simulink model "pv_battery_converter_simulation"  (Simulink 8.8)
settings: Solver=ode45  StartTime=0.0  StopTime=3600*14  FixedStep=0.01  RelTol=1e-3  EnableMultiTasking=on
undefined symbols (not defined in the file): G_vec, Ppv_to_Ipv, Ppv_vec
libraries: simulink x2
settings Model: LogicAnalyzerSignalOrdering=50bcff72-ad36-4fbe-b64f-51c65f6cd540,5d435876-f604-47e5-bfe3-cb9cb4b23e1d,6b0e0226-71fb-4e57-ad2a-fabfdac615dd,e2076062-044c-4264-af36-cff1764121ec,6ceae382-cfb6-4c2b-9ce8-e51f041ad3d8,832e4e12-eea1-4e74-bd4f-841bea17a355,4353c241-6b25-4e3c-9a1f-18ea053f432e  SuppressorTable=22 serialization::archive 11 0 3 0 0 0 0 0  Creator=dhshin  LastModifiedBy=Robert
settings OptimizationCC: ExpressionDepthLimit=2147483647
settings DebuggingCC: SolverPrmCheckMsg=warning

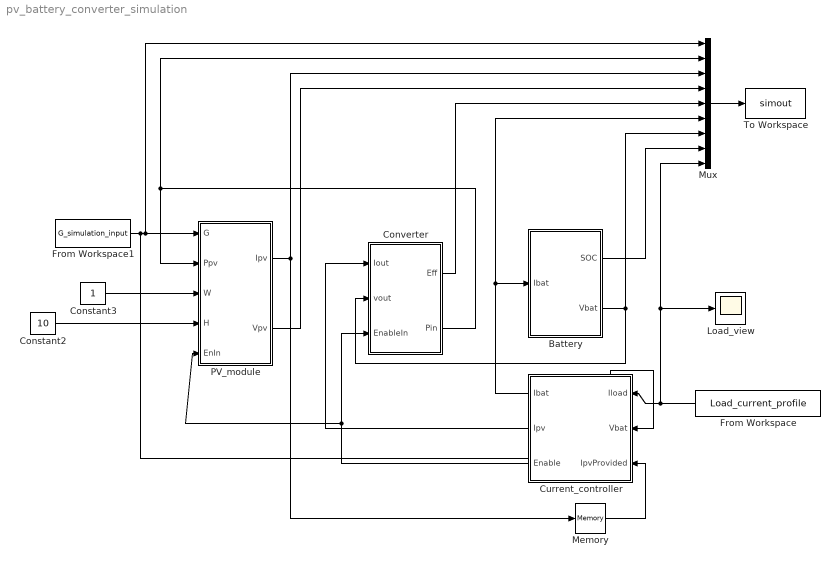
== system pv_battery_converter_simulation ==
  Battery : Subsystem
  Constant2 : Constant  Value=10
  Constant3 : Constant
  Converter : Subsystem
  Current_controller : Subsystem
  From Workspace : FromWorkspace  VariableName=Load_current_profile  SampleTime=0
  From Workspace1 : FromWorkspace  VariableName=G_simulation_input  SampleTime=0
  Load_view : Scope
  Memory : Memory
  Mux : Mux  Inputs=9
  PV_module : Subsystem
  To Workspace : ToWorkspace  VariableName=simout  SaveFormat=Structure  SampleTime=-1
  wires:
  From Workspace1/1 -> PV_module/1(G), Mux/1, Current_controller/2(Vbat)
  Mux/1 -> To Workspace/1
  Constant2/1 -> PV_module/4(H)
  Constant3/1 -> PV_module/3(W)
  From Workspace/1 -> Current_controller/1(Iload), Mux/9, Load_view/1
  Current_controller/1(Ibat) -> Battery/1(Ibat), Mux/6
  Current_controller/2(Ipv) -> Converter/1(Iout)
  Battery/2(Vbat) -> Mux/7, Converter/2(vout)
  PV_module/2(Vpv) -> Mux/4
  Converter/2(Pin) -> PV_module/2(Ppv), Mux/2
  PV_module/1(Ipv) -> Mux/3, Memory/1
  Converter/1(Eff) -> Mux/5
  Battery/1(SOC) -> Mux/8
  Current_controller/3(Enable) -> PV_module/5(EnIn), Converter/3(EnableIn)
  Memory/1 -> Current_controller/3(IpvProvided)

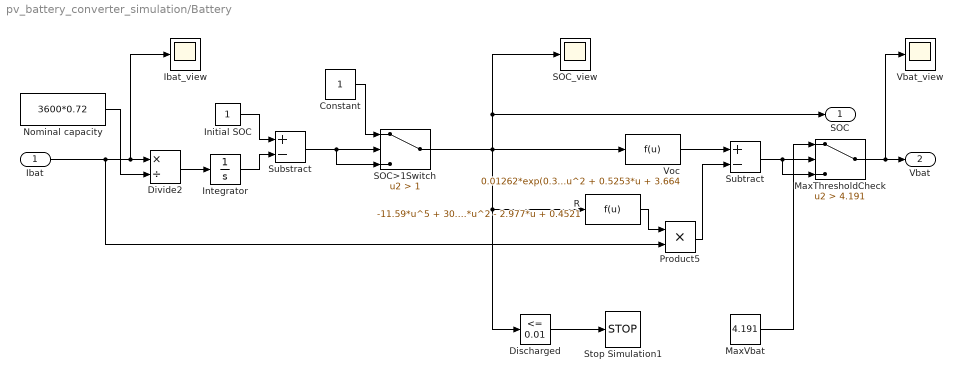
== system pv_battery_converter_simulation/Battery ==
  Ibat : Inport
  Constant : Constant
  Discharged : simulink/Logic and Bit Operations/Compare To Constant  relop=<=  const=0.01  OutDataTypeStr=boolean
  Divide2 : Product  Inputs=*/
  Ibat_view : Scope
  Initial SOC : Constant
  Integrator : Integrator
  MaxThresholdCheck : Switch  Criteria=u2 > Threshold  Threshold=4.191
  MaxVbat : Constant  Value=4.191
  Nominal capacity : Constant  Value=3600*0.72
  Product5 : Product  RndMeth=Zero
  R : Fcn  Expr=-11.59*u^5 + 30.82*u^4 - 30.55*u^3 + 13.97*u^2 - 2.977*u + 0.4521
  "SOC>1Switch " : Switch  Criteria=u2 > Threshold  Threshold=1
  SOC_view : Scope
  Stop Simulation1 : Stop
  Substract : Sum  Inputs=+-
  Subtract : Sum  Inputs=+-
  Vbat_view : Scope
  Voc : Fcn  Expr=0.01262*exp(0.3703*u) + 0.1237*u^4 + 0.14*u^3 - 0.2619*u^2 + 0.5253*u + 3.664
  SOC : Outport
  Vbat : Outport  Port=2
  wires:
  Ibat/1 -> Product5/2, Divide2/1, Ibat_view/1
  Product5/1 -> Subtract/2
  Subtract/1 -> MaxThresholdCheck/3, MaxThresholdCheck/2
  R/1 -> Product5/1
  Voc/1 -> Subtract/1
  Nominal capacity/1 -> Divide2/2
  Divide2/1 -> Integrator/1
  Integrator/1 -> Substract/2
  Initial SOC/1 -> Substract/1
  Discharged/1 -> Stop Simulation1/1
  Constant/1 -> "SOC>1Switch "/1
  Substract/1 -> "SOC>1Switch "/2, "SOC>1Switch "/3
  "SOC>1Switch "/1 -> SOC/1, SOC_view/1, Discharged/1, R/1, Voc/1
  MaxVbat/1 -> MaxThresholdCheck/1
  MaxThresholdCheck/1 -> Vbat_view/1, Vbat/1

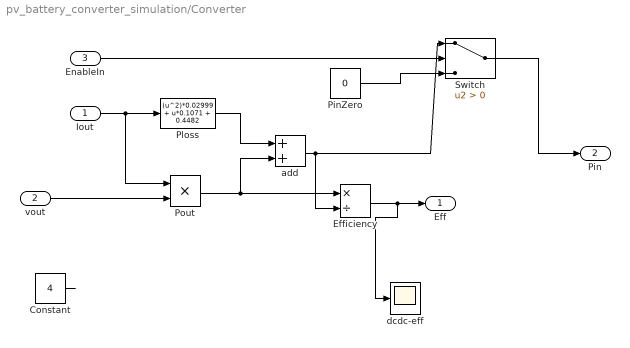
== system pv_battery_converter_simulation/Converter ==
  Iout : Inport
  vout : Inport  Port=2
  EnableIn : Inport  Port=3
  Constant : Constant  Value=4
  Efficiency : Product  Inputs=*/
  PinZero : Constant  Value=0
  Ploss : Fcn  Expr=(u^2)*0.02999 + u*0.1071 + 0.4482
  Pout : Product  RndMeth=Zero
  Switch : Switch  Criteria=u2 > Threshold
  add : Sum
  "dcdc-eff " : Scope
  Eff : Outport
  Pin : Outport  Port=2
  wires:
  Iout/1 -> Ploss/1, Pout/1
  vout/1 -> Pout/2
  Ploss/1 -> add/1
  Pout/1 -> add/2, Efficiency/1
  add/1 -> Switch/1, Efficiency/2
  Efficiency/1 -> "dcdc-eff "/1, Eff/1
  EnableIn/1 -> Switch/2
  Switch/1 -> Pin/1
  PinZero/1 -> Switch/3
  Constant/1 -> ?

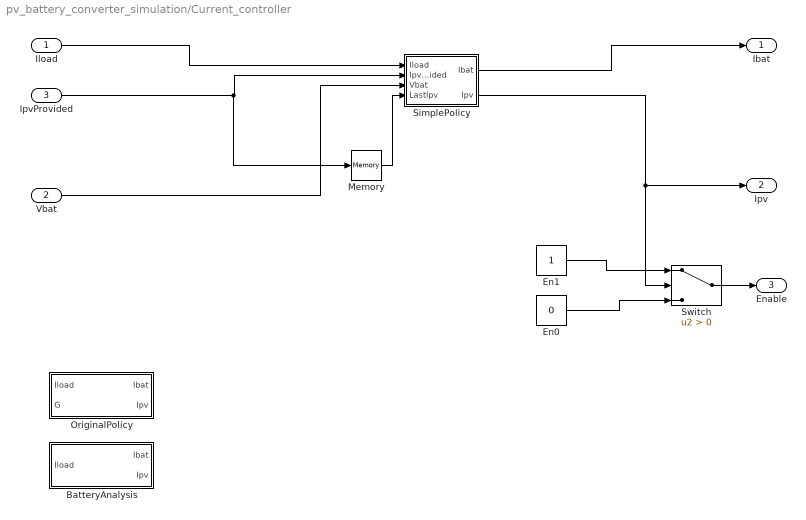
== system pv_battery_converter_simulation/Current_controller ==
  Iload : Inport
  Vbat : Inport  Port=2
  IpvProvided : Inport  Port=3
  "BatteryAnalysis " : Subsystem  TreatAsAtomicUnit=on
      settings: RTWFcnNameOpts=Use subsystem name  RTWFileNameOpts=Use function name
  En0 : Constant  Value=0
  En1 : Constant
  Memory : Memory
  OriginalPolicy : Subsystem  TreatAsAtomicUnit=on
      settings: RTWFcnNameOpts=Use subsystem name  RTWFileNameOpts=Use function name
  "SimplePolicy " : MATLAB Function  TreatAsAtomicUnit=on
  Switch : Switch  Criteria=u2 > Threshold
  Ibat : Outport
  Ipv : Outport  Port=2
  Enable : Outport  Port=3
  wires:
  Vbat/1 -> "SimplePolicy "/3(Vbat)
  Iload/1 -> "SimplePolicy "/1(Iload)
  "SimplePolicy "/1(Ibat) -> Ibat/1
  "SimplePolicy "/2(Ipv) -> Switch/2, Ipv/1
  En1/1 -> Switch/1
  En0/1 -> Switch/3
  Switch/1 -> Enable/1
  IpvProvided/1 -> Memory/1, "SimplePolicy "/2(IpvProvided)
  Memory/1 -> "SimplePolicy "/4(LastIpv)

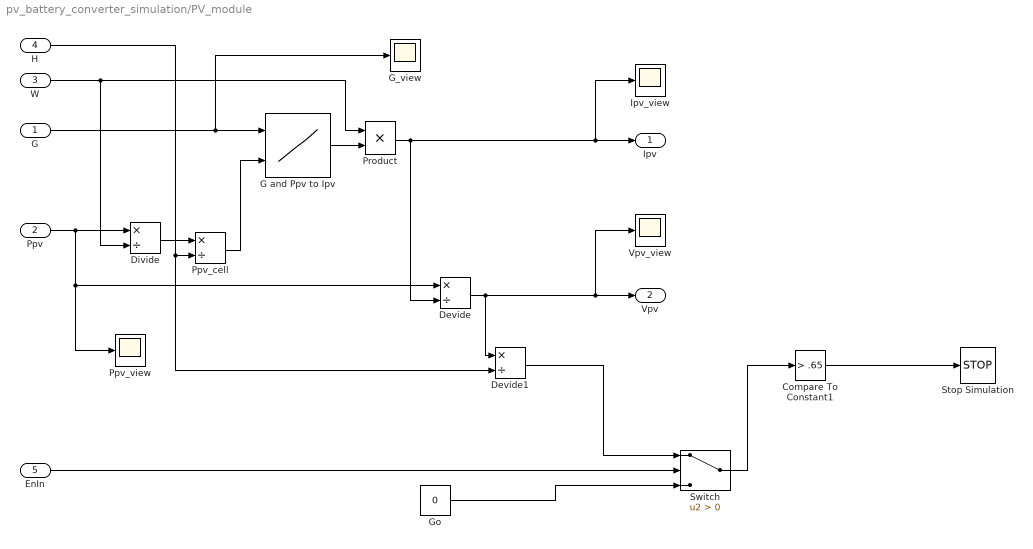
== system pv_battery_converter_simulation/PV_module ==
  G : Inport
  Ppv : Inport  Port=2
  W : Inport  Port=3
  H : Inport  Port=4
  EnIn : Inport  Port=5
  Compare To Constant1 : simulink/Logic and Bit Operations/Compare To Constant  relop=>  const=.65  OutDataTypeStr=boolean  ZeroCross=off
  Devide : Product  Inputs=*/
  Devide1 : Product  Inputs=*/
  Divide : Product  Inputs=*/
  G and Ppv to Ipv : Lookup_n-D  BreakpointsForDimension1=G_vec  BreakpointsForDimension2=Ppv_vec  Table=Ppv_to_Ipv  RndMeth=Simplest  InputSameDT=on
  G_view : Scope
  Go : Constant  Value=0
  Ipv_view : Scope
  Ppv_cell : Product  Inputs=*/
  Ppv_view : Scope
  Product : Product  RndMeth=Zero
  Stop Simulation : Stop
  Switch : Switch  Criteria=u2 > Threshold
  Vpv_view : Scope
  Ipv : Outport
  Vpv : Outport  Port=2
  wires:
  G/1 -> G and Ppv to Ipv/1, G_view/1
  G and Ppv to Ipv/1 -> Product/2
  Product/1 -> Devide/2, Ipv_view/1, Ipv/1
  Ppv/1 -> Divide/1, Devide/1, Ppv_view/1
  Ppv_cell/1 -> G and Ppv to Ipv/2
  Divide/1 -> Ppv_cell/1
  W/1 -> Divide/2, Product/1
  H/1 -> Ppv_cell/2, Devide1/2
  Devide/1 -> Vpv/1, Vpv_view/1, Devide1/1
  Devide1/1 -> Switch/1
  Compare To Constant1/1 -> Stop Simulation/1
  Go/1 -> Switch/3
  EnIn/1 -> Switch/2
  Switch/1 -> Compare To Constant1/1

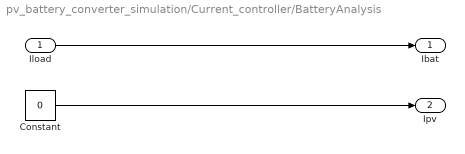
== system pv_battery_converter_simulation/Current_controller/BatteryAnalysis  ==
  Iload : Inport
  Constant : Constant  Value=0
  Ibat : Outport
  Ipv : Outport  Port=2
  wires:
  Iload/1 -> Ibat/1
  Constant/1 -> Ipv/1

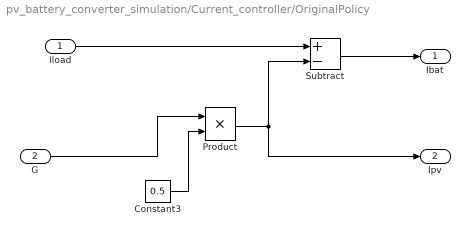
== system pv_battery_converter_simulation/Current_controller/OriginalPolicy ==
  Iload : Inport
  G : Inport  Port=2
  Constant3 : Constant  Value=0.5
  Product : Product  RndMeth=Zero
  Subtract : Sum  Inputs=+-
  Ibat : Outport
  Ipv : Outport  Port=2
  wires:
  G/1 -> Product/1
  Constant3/1 -> Product/2
  Iload/1 -> Subtract/1
  Subtract/1 -> Ibat/1
  Product/1 -> Ipv/1, Subtract/2

== matlab function Current_controller/SimplePolicy  ==
  data: Iload input double; Ibat output double; Ipv output double; IpvProvided input double; Vbat input double; LastIpv input double
function [Ibat, Ipv] = fcn(Iload, IpvProvided, Vbat, LastIpv)
    if Iload < 0.5*IpvProvided   % delegate the work to the pv panel and...
        if IpvProvided > LastIpv   % G is increasing, ask all to the pv panel (none to the battery)
            Ipv = Iload;
            if Vbat < 4.0    % max Vbat is 4.191
                Ibat = Iload - 0.5*IpvProvided; % recharge the battery ...
            else
                Ibat = 0;
            end
        else   % G is decreasing, ask less from the pv panel
            Ipv = 0.7*Iload;
            Ibat = 0.3*Iload;
        end
    else   % delegate the work fully to the battery
            Ibat =  Iload;
            Ipv = 0;
    end
